simulink model "RealLifeTrainModel"  (R2024a)
settings: Solver=ode1  StartTime=0.0  StopTime=Inf  FixedStep=0.001  RelTol=1e-3
PostLoadFcn:
  | , if any(exist('dsrtsu_mdlpostloadfcn', 'file') ~= 0), dsrtsu_mdlpostloadfcn('Execute', bdroot); end,
InitFcn:
  | , if any(exist('rtifpga_mdlclblib', 'file') ~= 0), rtifpga_mdlclblib('Init', bdroot); end,
undefined symbols (not defined in the file): DiscIntNeverNeededParam
libraries: deeplib x29, svdutilitieslib x28, simulink x8, eeGeneralControl x8, rti1202lib_adc_class1 x6, rti1202serlib x5, spsEdgeDetectorLib x5, rtiemclib x2, rti1202lib_dac_class1 x1
(part 4 of 8)

== system RealLifeTrainModel/ContractionMetricFilterSystem3/Mdot_subsystem/IndidualGrad2 ==
  State : Inport
  Position : Inport  Port=2
  StartValue : Inport  Port=3
  ConvertMatrix : MATLAB Function  TreatAsAtomicUnit=on
  Data Type Conversion1 : DataTypeConversion  OutDataTypeStr=single  SaturateOnIntegerOverflow=off  RndMeth=Floor
  Data Type Conversion2 : DataTypeConversion  OutDataTypeStr=single  SaturateOnIntegerOverflow=off  RndMeth=Floor
  MATLAB Function2 : MATLAB Function  TreatAsAtomicUnit=on
  MATLAB Function5 : MATLAB Function  TreatAsAtomicUnit=on
  PredictMetric : deeplib/Predict  Network=Network from MAT-file  NetworkFunction=squeezenet  NetworkFilePath=C:\Users\ic2d\Documents\GitHub\dSpace_Controllers_legged\metric.mat  MiniBatchSize=128  InputDataFormats={'input', 'BC';}  Predictions=on  Activations={}  ForceInterpretedSim=off  EnableDLNetwork=on  LastKnownNetworkFilePath='C:\Users\ic2d\Documents\GitHub\dSpace_Controllers_legged\metric.mat'  LastKnownNetworkTimeStamp=739864.429490740760229527950286865234375
  Sum4 : Sum  Inputs=|++
  Grad : Outport
  wires:
  Sum4/1 -> Data Type Conversion2/1
  StartValue/1 -> MATLAB Function5/2(u2)
  Data Type Conversion1/1 -> ConvertMatrix/1(M_flat)
  [GradConst] -> MATLAB Function5/3(const)
  PredictMetric/1 -> Data Type Conversion1/1
  MATLAB Function5/1(y) -> Grad/1
  Position/1 -> MATLAB Function2/2(pos)
  [GradConst] -> MATLAB Function2/1(u)
  MATLAB Function2/1(y) -> Sum4/2
  State/1 -> Sum4/1
  Data Type Conversion2/1 -> PredictMetric/1
  ConvertMatrix/1(M) -> MATLAB Function5/1(u1)

== system RealLifeTrainModel/ContractionMetricFilterSystem3/Mdot_subsystem/IndidualGrad3 ==
  State : Inport
  Position : Inport  Port=2
  StartValue : Inport  Port=3
  ConvertMatrix : MATLAB Function  TreatAsAtomicUnit=on
  Data Type Conversion1 : DataTypeConversion  OutDataTypeStr=single  SaturateOnIntegerOverflow=off  RndMeth=Floor
  Data Type Conversion2 : DataTypeConversion  OutDataTypeStr=single  SaturateOnIntegerOverflow=off  RndMeth=Floor
  MATLAB Function2 : MATLAB Function  TreatAsAtomicUnit=on
  MATLAB Function5 : MATLAB Function  TreatAsAtomicUnit=on
  PredictMetric : deeplib/Predict  Network=Network from MAT-file  NetworkFunction=squeezenet  NetworkFilePath=C:\Users\ic2d\Documents\GitHub\dSpace_Controllers_legged\metric.mat  MiniBatchSize=128  InputDataFormats={'input', 'BC';}  Predictions=on  Activations={}  ForceInterpretedSim=off  EnableDLNetwork=on  LastKnownNetworkFilePath='C:\Users\ic2d\Documents\GitHub\dSpace_Controllers_legged\metric.mat'  LastKnownNetworkTimeStamp=739864.429490740760229527950286865234375
  Sum4 : Sum  Inputs=|++
  Grad : Outport
  wires:
  Sum4/1 -> Data Type Conversion2/1
  StartValue/1 -> MATLAB Function5/2(u2)
  Data Type Conversion1/1 -> ConvertMatrix/1(M_flat)
  [GradConst] -> MATLAB Function5/3(const)
  PredictMetric/1 -> Data Type Conversion1/1
  MATLAB Function5/1(y) -> Grad/1
  Position/1 -> MATLAB Function2/2(pos)
  [GradConst] -> MATLAB Function2/1(u)
  MATLAB Function2/1(y) -> Sum4/2
  State/1 -> Sum4/1
  Data Type Conversion2/1 -> PredictMetric/1
  ConvertMatrix/1(M) -> MATLAB Function5/1(u1)

== system RealLifeTrainModel/ContractionMetricFilterSystem3/Mdot_subsystem/IndidualGrad4 ==
  State : Inport
  Position : Inport  Port=2
  StartValue : Inport  Port=3
  ConvertMatrix : MATLAB Function  TreatAsAtomicUnit=on
  Data Type Conversion1 : DataTypeConversion  OutDataTypeStr=single  SaturateOnIntegerOverflow=off  RndMeth=Floor
  Data Type Conversion2 : DataTypeConversion  OutDataTypeStr=single  SaturateOnIntegerOverflow=off  RndMeth=Floor
  MATLAB Function2 : MATLAB Function  TreatAsAtomicUnit=on
  MATLAB Function5 : MATLAB Function  TreatAsAtomicUnit=on
  PredictMetric : deeplib/Predict  Network=Network from MAT-file  NetworkFunction=squeezenet  NetworkFilePath=C:\Users\ic2d\Documents\GitHub\dSpace_Controllers_legged\metric.mat  MiniBatchSize=128  InputDataFormats={'input', 'BC';}  Predictions=on  Activations={}  ForceInterpretedSim=off  EnableDLNetwork=on  LastKnownNetworkFilePath='C:\Users\ic2d\Documents\GitHub\dSpace_Controllers_legged\metric.mat'  LastKnownNetworkTimeStamp=739864.429490740760229527950286865234375
  Sum4 : Sum  Inputs=|++
  Grad : Outport
  wires:
  Sum4/1 -> Data Type Conversion2/1
  StartValue/1 -> MATLAB Function5/2(u2)
  Data Type Conversion1/1 -> ConvertMatrix/1(M_flat)
  [GradConst] -> MATLAB Function5/3(const)
  PredictMetric/1 -> Data Type Conversion1/1
  MATLAB Function5/1(y) -> Grad/1
  Position/1 -> MATLAB Function2/2(pos)
  [GradConst] -> MATLAB Function2/1(u)
  MATLAB Function2/1(y) -> Sum4/2
  State/1 -> Sum4/1
  Data Type Conversion2/1 -> PredictMetric/1
  ConvertMatrix/1(M) -> MATLAB Function5/1(u1)

== system RealLifeTrainModel/ContractionMetricFilterSystem3/Mdot_subsystem/IndidualGrad5 ==
  State : Inport
  Position : Inport  Port=2
  StartValue : Inport  Port=3
  ConvertMatrix : MATLAB Function  TreatAsAtomicUnit=on
  Data Type Conversion1 : DataTypeConversion  OutDataTypeStr=single  SaturateOnIntegerOverflow=off  RndMeth=Floor
  Data Type Conversion2 : DataTypeConversion  OutDataTypeStr=single  SaturateOnIntegerOverflow=off  RndMeth=Floor
  MATLAB Function2 : MATLAB Function  TreatAsAtomicUnit=on
  MATLAB Function5 : MATLAB Function  TreatAsAtomicUnit=on
  PredictMetric : deeplib/Predict  Network=Network from MAT-file  NetworkFunction=squeezenet  NetworkFilePath=C:\Users\ic2d\Documents\GitHub\dSpace_Controllers_legged\metric.mat  MiniBatchSize=128  InputDataFormats={'input', 'BC';}  Predictions=on  Activations={}  ForceInterpretedSim=off  EnableDLNetwork=on  LastKnownNetworkFilePath='C:\Users\ic2d\Documents\GitHub\dSpace_Controllers_legged\metric.mat'  LastKnownNetworkTimeStamp=739864.429490740760229527950286865234375
  Sum4 : Sum  Inputs=|++
  Grad : Outport
  wires:
  Sum4/1 -> Data Type Conversion2/1
  StartValue/1 -> MATLAB Function5/2(u2)
  Data Type Conversion1/1 -> ConvertMatrix/1(M_flat)
  [GradConst] -> MATLAB Function5/3(const)
  PredictMetric/1 -> Data Type Conversion1/1
  MATLAB Function5/1(y) -> Grad/1
  Position/1 -> MATLAB Function2/2(pos)
  [GradConst] -> MATLAB Function2/1(u)
  MATLAB Function2/1(y) -> Sum4/2
  State/1 -> Sum4/1
  Data Type Conversion2/1 -> PredictMetric/1
  ConvertMatrix/1(M) -> MATLAB Function5/1(u1)

== system RealLifeTrainModel/ContractionMetricFilterSystem3/Mdot_subsystem/IndidualGrad6 ==
  State : Inport
  Position : Inport  Port=2
  StartValue : Inport  Port=3
  ConvertMatrix : MATLAB Function  TreatAsAtomicUnit=on
  Data Type Conversion1 : DataTypeConversion  OutDataTypeStr=single  SaturateOnIntegerOverflow=off  RndMeth=Floor
  Data Type Conversion2 : DataTypeConversion  OutDataTypeStr=single  SaturateOnIntegerOverflow=off  RndMeth=Floor
  MATLAB Function2 : MATLAB Function  TreatAsAtomicUnit=on
  MATLAB Function5 : MATLAB Function  TreatAsAtomicUnit=on
  PredictMetric : deeplib/Predict  Network=Network from MAT-file  NetworkFunction=squeezenet  NetworkFilePath=C:\Users\ic2d\Documents\GitHub\dSpace_Controllers_legged\metric.mat  MiniBatchSize=128  InputDataFormats={'input', 'BC';}  Predictions=on  Activations={}  ForceInterpretedSim=off  EnableDLNetwork=on  LastKnownNetworkFilePath='C:\Users\ic2d\Documents\GitHub\dSpace_Controllers_legged\metric.mat'  LastKnownNetworkTimeStamp=739864.429490740760229527950286865234375
  Sum4 : Sum  Inputs=|++
  Grad : Outport
  wires:
  Sum4/1 -> Data Type Conversion2/1
  StartValue/1 -> MATLAB Function5/2(u2)
  Data Type Conversion1/1 -> ConvertMatrix/1(M_flat)
  [GradConst] -> MATLAB Function5/3(const)
  PredictMetric/1 -> Data Type Conversion1/1
  MATLAB Function5/1(y) -> Grad/1
  Position/1 -> MATLAB Function2/2(pos)
  [GradConst] -> MATLAB Function2/1(u)
  MATLAB Function2/1(y) -> Sum4/2
  State/1 -> Sum4/1
  Data Type Conversion2/1 -> PredictMetric/1
  ConvertMatrix/1(M) -> MATLAB Function5/1(u1)

== system RealLifeTrainModel/ContractionMetricFilterSystem3/Mdot_subsystem/IndidualGrad7 ==
  State : Inport
  Position : Inport  Port=2
  StartValue : Inport  Port=3
  ConvertMatrix : MATLAB Function  TreatAsAtomicUnit=on
  Data Type Conversion1 : DataTypeConversion  OutDataTypeStr=single  SaturateOnIntegerOverflow=off  RndMeth=Floor
  Data Type Conversion2 : DataTypeConversion  OutDataTypeStr=single  SaturateOnIntegerOverflow=off  RndMeth=Floor
  MATLAB Function2 : MATLAB Function  TreatAsAtomicUnit=on
  MATLAB Function5 : MATLAB Function  TreatAsAtomicUnit=on
  PredictMetric : deeplib/Predict  Network=Network from MAT-file  NetworkFunction=squeezenet  NetworkFilePath=C:\Users\ic2d\Documents\GitHub\dSpace_Controllers_legged\metric.mat  MiniBatchSize=128  InputDataFormats={'input', 'BC';}  Predictions=on  Activations={}  ForceInterpretedSim=off  EnableDLNetwork=on  LastKnownNetworkFilePath='C:\Users\ic2d\Documents\GitHub\dSpace_Controllers_legged\metric.mat'  LastKnownNetworkTimeStamp=739864.429490740760229527950286865234375
  Sum4 : Sum  Inputs=|++
  Grad : Outport
  wires:
  Sum4/1 -> Data Type Conversion2/1
  StartValue/1 -> MATLAB Function5/2(u2)
  Data Type Conversion1/1 -> ConvertMatrix/1(M_flat)
  [GradConst] -> MATLAB Function5/3(const)
  PredictMetric/1 -> Data Type Conversion1/1
  MATLAB Function5/1(y) -> Grad/1
  Position/1 -> MATLAB Function2/2(pos)
  [GradConst] -> MATLAB Function2/1(u)
  MATLAB Function2/1(y) -> Sum4/2
  State/1 -> Sum4/1
  Data Type Conversion2/1 -> PredictMetric/1
  ConvertMatrix/1(M) -> MATLAB Function5/1(u1)

== system RealLifeTrainModel/RTI Data/RTI Data Store/RTI Data Store ==
  RTI Data Store : Subsystem  mask(RTI_DATA_STORE){}
      mask help:
      | RTI Data Store Block. This block is used by RTI to store internal model dependent data. Deleting this block will result in data loss.
      |
      | NEVER DELETE, COPY, OR MODIFY THIS BLOCK!
      mask Help:
      | RTI Data Store Block. This block is used by RTI to store internal model dependent data. Deleting this block will result in data loss.
      | 
      | NEVER DELETE, COPY, OR MODIFY THIS BLOCK!
      mask Display: text(0.5, 0.5, ' ', 'HorizontalAlignment', 'center');

== system RealLifeTrainModel/CommSystem/SendMessageSystem/CancelSubsystem/If Action Subsystem ==
  Action Port : ActionPort  ActionPortLabel=if(u1 > 0)
  Cast : DataTypeConversion  OutDataTypeStr=double  SaturateOnIntegerOverflow=off  RndMeth=Floor
  Cast1 : DataTypeConversion  OutDataTypeStr=double  SaturateOnIntegerOverflow=off  RndMeth=Floor
  Constant : Constant  Value=0  OutDataTypeStr=uint8
  Data Store Write : DataStoreWrite  DataStoreName=FlagAbort  IndexOptions=Index vector (dialog)  Indices=1  OutputSizes=1
  Data Store Write2 : DataStoreWrite  DataStoreName=FlagStartTrain  IndexOptions=Index vector (dialog)  Indices=1  OutputSizes=1
  Data Store Write3 : DataStoreWrite  DataStoreName=OutputReceived  IndexOptions=Index vector (dialog)  Indices=1  OutputSizes=1
  Data Store Write4 : DataStoreWrite  DataStoreName=StartSignalValue  IndexOptions=Index vector (dialog)  Indices=1  OutputSizes=1
  wires:
  Constant/1 -> Cast1/1, Cast/1, Data Store Write2/1, Data Store Write/1
  Cast1/1 -> Data Store Write3/1
  Cast/1 -> Data Store Write4/1

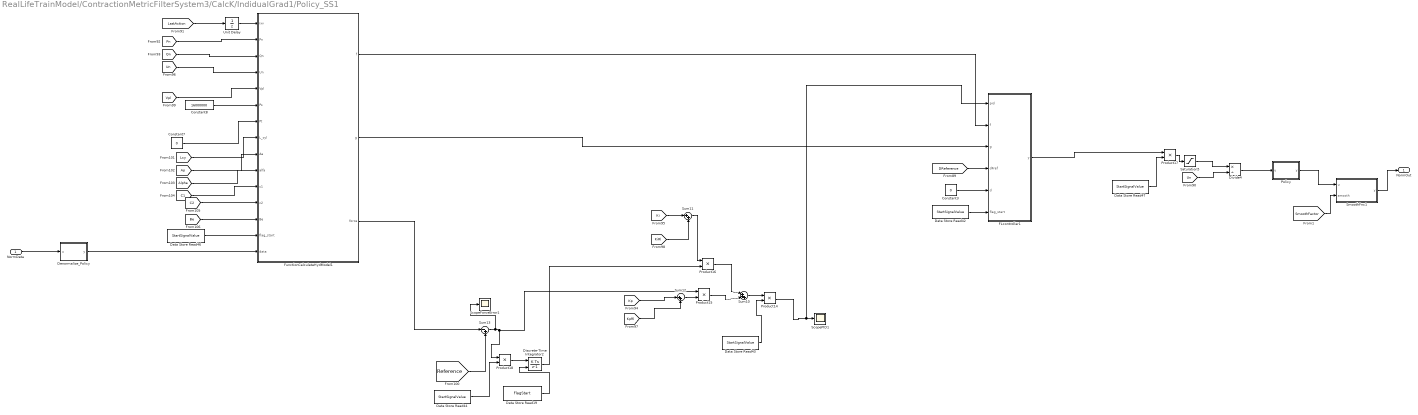
== system RealLifeTrainModel/ContractionMetricFilterSystem3/CalcK/IndidualGrad1/Policy_SS1 ==
  NormData : Inport
  Constant3 : Constant  Value=0
  Constant7 : Constant  Value=0
  Constant8 : Constant  Value=16000000
  Data Store Read19 : DataStoreRead  DataStoreName=FlagStart  IndexOptions=Index vector (dialog)  Indices=1  OutputSizes=1
  Data Store Read{42..44,46..47} (5 alike) : DataStoreRead  DataStoreName=StartSignalValue  IndexOptions=Index vector (dialog)  Indices=1  OutputSizes=1
  Denormalize_Policy : MATLAB Function  TreatAsAtomicUnit=on
  Discrete-Time Integrator2 : DiscreteIntegrator  ExternalReset=either  SampleTime=-1  ICPrevOutput=DiscIntNeverNeededParam  ICPrevScaledInput=DiscIntNeverNeededParam
  Divide4 : Product  Inputs=*/
  FLcontroller1 : MATLAB Function  TreatAsAtomicUnit=on
  FunctionCalculateHydModel1 : MATLAB Function  TreatAsAtomicUnit=on
  Policy : MATLAB Function  TreatAsAtomicUnit=on
  Product{14..18} (5 alike) : Product
  Saturation5 : Saturate  UpperLimit=str2num(get_param('Teste_PID/Un','Value'))/str2num(get_param('Teste_PID/SaturationDivider','Value'))  LowerLimit=-str2num(get_param('Teste_PID/Un','Value'))/str2num(get_param('Teste_PID/SaturationDivider','Value'))
  ScopeForceError1 : Scope
  ScopePID1 : Scope
  SmoothFnc1 : MATLAB Function  TreatAsAtomicUnit=on
  Sum10 : Sum  Inputs=|+++
  Sum11 : Sum  Inputs=|++
  Sum12 : Sum  Inputs=|++
  Sum13 : Sum  Inputs=|-+
  Unit Delay : UnitDelay  SampleTime=-1  HasFrameUpgradeWarning=on
  NormOut : Outport
  wires:
  FunctionCalculateHydModel1/3(force) -> Sum13/1
  [Vpl] -> FunctionCalculateHydModel1/5(Vpl)
  Sum13/1 -> ScopeForceError1/1, Product15/1, Product18/1
  [Alpha] -> FunctionCalculateHydModel1/10(alfa)
  [C2] -> FunctionCalculateHydModel1/12(c2)
  Data Store Read42/1 -> FLcontroller1/6(flag_start)
  [Be] -> FunctionCalculateHydModel1/13(Be)
  [Lcy] -> FunctionCalculateHydModel1/8(L_cyl)
  Data Store Read43/1 -> Product14/2
  [Ap] -> FunctionCalculateHydModel1/9(Aa)
  Product15/1 -> Sum10/2
  Data Store Read44/1 -> Product18/2
  Product18/1 -> Discrete-Time Integrator2/1
  [KpRl] -> Sum12/2
  [Reference] -> Sum13/2
  Constant8/1 -> FunctionCalculateHydModel1/6(Ps)
  Product14/1 -> FLcontroller1/1(pid), ScopePID1/1
  Sum11/1 -> Product16/1
  Sum12/1 -> Product15/2
  Saturation5/1 -> Divide4/1
  [Un] -> Divide4/2
  FLcontroller1/1(y) -> Product17/1
  Denormalize_Policy/1(y) -> FunctionCalculateHydModel1/15(data)
  Sum10/1 -> Product14/1
  [C1] -> FunctionCalculateHydModel1/11(c1)
  Discrete-Time Integrator2/1 -> Product16/2
  [Pn] -> FunctionCalculateHydModel1/2(Pn)
  [LastAction] -> Unit Delay/1
  [Kp] -> Sum12/1
  [Ki] -> Sum11/1
  Constant7/1 -> FunctionCalculateHydModel1/7(Pt)
  Divide4/1 -> Policy/1(u)
  [Qn] -> FunctionCalculateHydModel1/3(Qn)
  Constant3/1 -> FLcontroller1/5(d)
  [KiRl] -> Sum11/2
  Data Store Read47/1 -> Product17/2
  Product16/1 -> Sum10/1
  FunctionCalculateHydModel1/2(g) -> FLcontroller1/3(g)
  Product17/1 -> Saturation5/1
  [DReference] -> FLcontroller1/4(dFref)
  FunctionCalculateHydModel1/1(f) -> FLcontroller1/2(f)
  [Un] -> FunctionCalculateHydModel1/4(Un)
  Data Store Read46/1 -> FunctionCalculateHydModel1/14(flag_start)
  NormData/1 -> Denormalize_Policy/1(u)
  Unit Delay/1 -> FunctionCalculateHydModel1/1(ixv)
  SmoothFnc1/1(y) -> NormOut/1
  Policy/1(y) -> SmoothFnc1/1(u)
  [SmoothFactor] -> SmoothFnc1/2(smooth)
  Data Store Read19/1 -> Discrete-Time Integrator2/2

== system RealLifeTrainModel/ContractionMetricFilterSystem3/CalcK/IndidualGrad10/Policy_SS1 ==
  NormData : Inport
  Constant3 : Constant  Value=0
  Constant7 : Constant  Value=0
  Constant8 : Constant  Value=16000000
  Data Store Read19 : DataStoreRead  DataStoreName=FlagStart  IndexOptions=Index vector (dialog)  Indices=1  OutputSizes=1
  Data Store Read{42..44,46..47} (5 alike) : DataStoreRead  DataStoreName=StartSignalValue  IndexOptions=Index vector (dialog)  Indices=1  OutputSizes=1
  Denormalize_Policy : MATLAB Function  TreatAsAtomicUnit=on
  Discrete-Time Integrator2 : DiscreteIntegrator  ExternalReset=either  SampleTime=-1  ICPrevOutput=DiscIntNeverNeededParam  ICPrevScaledInput=DiscIntNeverNeededParam
  Divide4 : Product  Inputs=*/
  FLcontroller1 : MATLAB Function  TreatAsAtomicUnit=on
  FunctionCalculateHydModel1 : MATLAB Function  TreatAsAtomicUnit=on
  Policy : MATLAB Function  TreatAsAtomicUnit=on
  Product{14..18} (5 alike) : Product
  Saturation5 : Saturate  UpperLimit=str2num(get_param('Teste_PID/Un','Value'))/str2num(get_param('Teste_PID/SaturationDivider','Value'))  LowerLimit=-str2num(get_param('Teste_PID/Un','Value'))/str2num(get_param('Teste_PID/SaturationDivider','Value'))
  ScopeForceError1 : Scope
  ScopePID1 : Scope
  SmoothFnc1 : MATLAB Function  TreatAsAtomicUnit=on
  Sum10 : Sum  Inputs=|+++
  Sum11 : Sum  Inputs=|++
  Sum12 : Sum  Inputs=|++
  Sum13 : Sum  Inputs=|-+
  Unit Delay : UnitDelay  SampleTime=-1  HasFrameUpgradeWarning=on
  NormOut : Outport
  wires:
  FunctionCalculateHydModel1/3(force) -> Sum13/1
  [Vpl] -> FunctionCalculateHydModel1/5(Vpl)
  Sum13/1 -> ScopeForceError1/1, Product15/1, Product18/1
  [Alpha] -> FunctionCalculateHydModel1/10(alfa)
  [C2] -> FunctionCalculateHydModel1/12(c2)
  Data Store Read42/1 -> FLcontroller1/6(flag_start)
  [Be] -> FunctionCalculateHydModel1/13(Be)
  [Lcy] -> FunctionCalculateHydModel1/8(L_cyl)
  Data Store Read43/1 -> Product14/2
  [Ap] -> FunctionCalculateHydModel1/9(Aa)
  Product15/1 -> Sum10/2
  Data Store Read44/1 -> Product18/2
  Product18/1 -> Discrete-Time Integrator2/1
  [KpRl] -> Sum12/2
  [Reference] -> Sum13/2
  Constant8/1 -> FunctionCalculateHydModel1/6(Ps)
  Product14/1 -> FLcontroller1/1(pid), ScopePID1/1
  Sum11/1 -> Product16/1
  Sum12/1 -> Product15/2
  Saturation5/1 -> Divide4/1
  [Un] -> Divide4/2
  FLcontroller1/1(y) -> Product17/1
  Denormalize_Policy/1(y) -> FunctionCalculateHydModel1/15(data)
  Sum10/1 -> Product14/1
  [C1] -> FunctionCalculateHydModel1/11(c1)
  Discrete-Time Integrator2/1 -> Product16/2
  [Pn] -> FunctionCalculateHydModel1/2(Pn)
  [LastAction] -> Unit Delay/1
  [Kp] -> Sum12/1
  [Ki] -> Sum11/1
  Constant7/1 -> FunctionCalculateHydModel1/7(Pt)
  Divide4/1 -> Policy/1(u)
  [Qn] -> FunctionCalculateHydModel1/3(Qn)
  Constant3/1 -> FLcontroller1/5(d)
  [KiRl] -> Sum11/2
  Data Store Read47/1 -> Product17/2
  Product16/1 -> Sum10/1
  FunctionCalculateHydModel1/2(g) -> FLcontroller1/3(g)
  Product17/1 -> Saturation5/1
  [DReference] -> FLcontroller1/4(dFref)
  FunctionCalculateHydModel1/1(f) -> FLcontroller1/2(f)
  [Un] -> FunctionCalculateHydModel1/4(Un)
  Data Store Read46/1 -> FunctionCalculateHydModel1/14(flag_start)
  NormData/1 -> Denormalize_Policy/1(u)
  Unit Delay/1 -> FunctionCalculateHydModel1/1(ixv)
  SmoothFnc1/1(y) -> NormOut/1
  Policy/1(y) -> SmoothFnc1/1(u)
  [SmoothFactor] -> SmoothFnc1/2(smooth)
  Data Store Read19/1 -> Discrete-Time Integrator2/2

== system RealLifeTrainModel/ContractionMetricFilterSystem3/CalcK/IndidualGrad2/Policy_SS1 ==
  NormData : Inport
  Constant3 : Constant  Value=0
  Constant7 : Constant  Value=0
  Constant8 : Constant  Value=16000000
  Data Store Read19 : DataStoreRead  DataStoreName=FlagStart  IndexOptions=Index vector (dialog)  Indices=1  OutputSizes=1
  Data Store Read{42..44,46..47} (5 alike) : DataStoreRead  DataStoreName=StartSignalValue  IndexOptions=Index vector (dialog)  Indices=1  OutputSizes=1
  Denormalize_Policy : MATLAB Function  TreatAsAtomicUnit=on
  Discrete-Time Integrator2 : DiscreteIntegrator  ExternalReset=either  SampleTime=-1  ICPrevOutput=DiscIntNeverNeededParam  ICPrevScaledInput=DiscIntNeverNeededParam
  Divide4 : Product  Inputs=*/
  FLcontroller1 : MATLAB Function  TreatAsAtomicUnit=on
  FunctionCalculateHydModel1 : MATLAB Function  TreatAsAtomicUnit=on
  Policy : MATLAB Function  TreatAsAtomicUnit=on
  Product{14..18} (5 alike) : Product
  Saturation5 : Saturate  UpperLimit=str2num(get_param('Teste_PID/Un','Value'))/str2num(get_param('Teste_PID/SaturationDivider','Value'))  LowerLimit=-str2num(get_param('Teste_PID/Un','Value'))/str2num(get_param('Teste_PID/SaturationDivider','Value'))
  ScopeForceError1 : Scope
  ScopePID1 : Scope
  SmoothFnc1 : MATLAB Function  TreatAsAtomicUnit=on
  Sum10 : Sum  Inputs=|+++
  Sum11 : Sum  Inputs=|++
  Sum12 : Sum  Inputs=|++
  Sum13 : Sum  Inputs=|-+
  Unit Delay : UnitDelay  SampleTime=-1  HasFrameUpgradeWarning=on
  NormOut : Outport
  wires:
  FunctionCalculateHydModel1/3(force) -> Sum13/1
  [Vpl] -> FunctionCalculateHydModel1/5(Vpl)
  Sum13/1 -> ScopeForceError1/1, Product15/1, Product18/1
  [Alpha] -> FunctionCalculateHydModel1/10(alfa)
  [C2] -> FunctionCalculateHydModel1/12(c2)
  Data Store Read42/1 -> FLcontroller1/6(flag_start)
  [Be] -> FunctionCalculateHydModel1/13(Be)
  [Lcy] -> FunctionCalculateHydModel1/8(L_cyl)
  Data Store Read43/1 -> Product14/2
  [Ap] -> FunctionCalculateHydModel1/9(Aa)
  Product15/1 -> Sum10/2
  Data Store Read44/1 -> Product18/2
  Product18/1 -> Discrete-Time Integrator2/1
  [KpRl] -> Sum12/2
  [Reference] -> Sum13/2
  Constant8/1 -> FunctionCalculateHydModel1/6(Ps)
  Product14/1 -> FLcontroller1/1(pid), ScopePID1/1
  Sum11/1 -> Product16/1
  Sum12/1 -> Product15/2
  Saturation5/1 -> Divide4/1
  [Un] -> Divide4/2
  FLcontroller1/1(y) -> Product17/1
  Denormalize_Policy/1(y) -> FunctionCalculateHydModel1/15(data)
  Sum10/1 -> Product14/1
  [C1] -> FunctionCalculateHydModel1/11(c1)
  Discrete-Time Integrator2/1 -> Product16/2
  [Pn] -> FunctionCalculateHydModel1/2(Pn)
  [LastAction] -> Unit Delay/1
  [Kp] -> Sum12/1
  [Ki] -> Sum11/1
  Constant7/1 -> FunctionCalculateHydModel1/7(Pt)
  Divide4/1 -> Policy/1(u)
  [Qn] -> FunctionCalculateHydModel1/3(Qn)
  Constant3/1 -> FLcontroller1/5(d)
  [KiRl] -> Sum11/2
  Data Store Read47/1 -> Product17/2
  Product16/1 -> Sum10/1
  FunctionCalculateHydModel1/2(g) -> FLcontroller1/3(g)
  Product17/1 -> Saturation5/1
  [DReference] -> FLcontroller1/4(dFref)
  FunctionCalculateHydModel1/1(f) -> FLcontroller1/2(f)
  [Un] -> FunctionCalculateHydModel1/4(Un)
  Data Store Read46/1 -> FunctionCalculateHydModel1/14(flag_start)
  NormData/1 -> Denormalize_Policy/1(u)
  Unit Delay/1 -> FunctionCalculateHydModel1/1(ixv)
  SmoothFnc1/1(y) -> NormOut/1
  Policy/1(y) -> SmoothFnc1/1(u)
  [SmoothFactor] -> SmoothFnc1/2(smooth)
  Data Store Read19/1 -> Discrete-Time Integrator2/2

== system RealLifeTrainModel/ContractionMetricFilterSystem3/CalcK/IndidualGrad3/Policy_SS1 ==
  NormData : Inport
  Constant3 : Constant  Value=0
  Constant7 : Constant  Value=0
  Constant8 : Constant  Value=16000000
  Data Store Read19 : DataStoreRead  DataStoreName=FlagStart  IndexOptions=Index vector (dialog)  Indices=1  OutputSizes=1
  Data Store Read{42..44,46..47} (5 alike) : DataStoreRead  DataStoreName=StartSignalValue  IndexOptions=Index vector (dialog)  Indices=1  OutputSizes=1
  Denormalize_Policy : MATLAB Function  TreatAsAtomicUnit=on
  Discrete-Time Integrator2 : DiscreteIntegrator  ExternalReset=either  SampleTime=-1  ICPrevOutput=DiscIntNeverNeededParam  ICPrevScaledInput=DiscIntNeverNeededParam
  Divide4 : Product  Inputs=*/
  FLcontroller1 : MATLAB Function  TreatAsAtomicUnit=on
  FunctionCalculateHydModel1 : MATLAB Function  TreatAsAtomicUnit=on
  Policy : MATLAB Function  TreatAsAtomicUnit=on
  Product{14..18} (5 alike) : Product
  Saturation5 : Saturate  UpperLimit=str2num(get_param('Teste_PID/Un','Value'))/str2num(get_param('Teste_PID/SaturationDivider','Value'))  LowerLimit=-str2num(get_param('Teste_PID/Un','Value'))/str2num(get_param('Teste_PID/SaturationDivider','Value'))
  ScopeForceError1 : Scope
  ScopePID1 : Scope
  SmoothFnc1 : MATLAB Function  TreatAsAtomicUnit=on
  Sum10 : Sum  Inputs=|+++
  Sum11 : Sum  Inputs=|++
  Sum12 : Sum  Inputs=|++
  Sum13 : Sum  Inputs=|-+
  Unit Delay : UnitDelay  SampleTime=-1  HasFrameUpgradeWarning=on
  NormOut : Outport
  wires:
  FunctionCalculateHydModel1/3(force) -> Sum13/1
  [Vpl] -> FunctionCalculateHydModel1/5(Vpl)
  Sum13/1 -> ScopeForceError1/1, Product15/1, Product18/1
  [Alpha] -> FunctionCalculateHydModel1/10(alfa)
  [C2] -> FunctionCalculateHydModel1/12(c2)
  Data Store Read42/1 -> FLcontroller1/6(flag_start)
  [Be] -> FunctionCalculateHydModel1/13(Be)
  [Lcy] -> FunctionCalculateHydModel1/8(L_cyl)
  Data Store Read43/1 -> Product14/2
  [Ap] -> FunctionCalculateHydModel1/9(Aa)
  Product15/1 -> Sum10/2
  Data Store Read44/1 -> Product18/2
  Product18/1 -> Discrete-Time Integrator2/1
  [KpRl] -> Sum12/2
  [Reference] -> Sum13/2
  Constant8/1 -> FunctionCalculateHydModel1/6(Ps)
  Product14/1 -> FLcontroller1/1(pid), ScopePID1/1
  Sum11/1 -> Product16/1
  Sum12/1 -> Product15/2
  Saturation5/1 -> Divide4/1
  [Un] -> Divide4/2
  FLcontroller1/1(y) -> Product17/1
  Denormalize_Policy/1(y) -> FunctionCalculateHydModel1/15(data)
  Sum10/1 -> Product14/1
  [C1] -> FunctionCalculateHydModel1/11(c1)
  Discrete-Time Integrator2/1 -> Product16/2
  [Pn] -> FunctionCalculateHydModel1/2(Pn)
  [LastAction] -> Unit Delay/1
  [Kp] -> Sum12/1
  [Ki] -> Sum11/1
  Constant7/1 -> FunctionCalculateHydModel1/7(Pt)
  Divide4/1 -> Policy/1(u)
  [Qn] -> FunctionCalculateHydModel1/3(Qn)
  Constant3/1 -> FLcontroller1/5(d)
  [KiRl] -> Sum11/2
  Data Store Read47/1 -> Product17/2
  Product16/1 -> Sum10/1
  FunctionCalculateHydModel1/2(g) -> FLcontroller1/3(g)
  Product17/1 -> Saturation5/1
  [DReference] -> FLcontroller1/4(dFref)
  FunctionCalculateHydModel1/1(f) -> FLcontroller1/2(f)
  [Un] -> FunctionCalculateHydModel1/4(Un)
  Data Store Read46/1 -> FunctionCalculateHydModel1/14(flag_start)
  NormData/1 -> Denormalize_Policy/1(u)
  Unit Delay/1 -> FunctionCalculateHydModel1/1(ixv)
  SmoothFnc1/1(y) -> NormOut/1
  Policy/1(y) -> SmoothFnc1/1(u)
  [SmoothFactor] -> SmoothFnc1/2(smooth)
  Data Store Read19/1 -> Discrete-Time Integrator2/2

== system RealLifeTrainModel/ContractionMetricFilterSystem3/CalcK/IndidualGrad4/Policy_SS1 ==
  NormData : Inport
  Constant3 : Constant  Value=0
  Constant7 : Constant  Value=0
  Constant8 : Constant  Value=16000000
  Data Store Read19 : DataStoreRead  DataStoreName=FlagStart  IndexOptions=Index vector (dialog)  Indices=1  OutputSizes=1
  Data Store Read{42..44,46..47} (5 alike) : DataStoreRead  DataStoreName=StartSignalValue  IndexOptions=Index vector (dialog)  Indices=1  OutputSizes=1
  Denormalize_Policy : MATLAB Function  TreatAsAtomicUnit=on
  Discrete-Time Integrator2 : DiscreteIntegrator  ExternalReset=either  SampleTime=-1  ICPrevOutput=DiscIntNeverNeededParam  ICPrevScaledInput=DiscIntNeverNeededParam
  Divide4 : Product  Inputs=*/
  FLcontroller1 : MATLAB Function  TreatAsAtomicUnit=on
  FunctionCalculateHydModel1 : MATLAB Function  TreatAsAtomicUnit=on
  Policy : MATLAB Function  TreatAsAtomicUnit=on
  Product{14..18} (5 alike) : Product
  Saturation5 : Saturate  UpperLimit=str2num(get_param('Teste_PID/Un','Value'))/str2num(get_param('Teste_PID/SaturationDivider','Value'))  LowerLimit=-str2num(get_param('Teste_PID/Un','Value'))/str2num(get_param('Teste_PID/SaturationDivider','Value'))
  ScopeForceError1 : Scope
  ScopePID1 : Scope
  SmoothFnc1 : MATLAB Function  TreatAsAtomicUnit=on
  Sum10 : Sum  Inputs=|+++
  Sum11 : Sum  Inputs=|++
  Sum12 : Sum  Inputs=|++
  Sum13 : Sum  Inputs=|-+
  Unit Delay : UnitDelay  SampleTime=-1  HasFrameUpgradeWarning=on
  NormOut : Outport
  wires:
  FunctionCalculateHydModel1/3(force) -> Sum13/1
  [Vpl] -> FunctionCalculateHydModel1/5(Vpl)
  Sum13/1 -> ScopeForceError1/1, Product15/1, Product18/1
  [Alpha] -> FunctionCalculateHydModel1/10(alfa)
  [C2] -> FunctionCalculateHydModel1/12(c2)
  Data Store Read42/1 -> FLcontroller1/6(flag_start)
  [Be] -> FunctionCalculateHydModel1/13(Be)
  [Lcy] -> FunctionCalculateHydModel1/8(L_cyl)
  Data Store Read43/1 -> Product14/2
  [Ap] -> FunctionCalculateHydModel1/9(Aa)
  Product15/1 -> Sum10/2
  Data Store Read44/1 -> Product18/2
  Product18/1 -> Discrete-Time Integrator2/1
  [KpRl] -> Sum12/2
  [Reference] -> Sum13/2
  Constant8/1 -> FunctionCalculateHydModel1/6(Ps)
  Product14/1 -> FLcontroller1/1(pid), ScopePID1/1
  Sum11/1 -> Product16/1
  Sum12/1 -> Product15/2
  Saturation5/1 -> Divide4/1
  [Un] -> Divide4/2
  FLcontroller1/1(y) -> Product17/1
  Denormalize_Policy/1(y) -> FunctionCalculateHydModel1/15(data)
  Sum10/1 -> Product14/1
  [C1] -> FunctionCalculateHydModel1/11(c1)
  Discrete-Time Integrator2/1 -> Product16/2
  [Pn] -> FunctionCalculateHydModel1/2(Pn)
  [LastAction] -> Unit Delay/1
  [Kp] -> Sum12/1
  [Ki] -> Sum11/1
  Constant7/1 -> FunctionCalculateHydModel1/7(Pt)
  Divide4/1 -> Policy/1(u)
  [Qn] -> FunctionCalculateHydModel1/3(Qn)
  Constant3/1 -> FLcontroller1/5(d)
  [KiRl] -> Sum11/2
  Data Store Read47/1 -> Product17/2
  Product16/1 -> Sum10/1
  FunctionCalculateHydModel1/2(g) -> FLcontroller1/3(g)
  Product17/1 -> Saturation5/1
  [DReference] -> FLcontroller1/4(dFref)
  FunctionCalculateHydModel1/1(f) -> FLcontroller1/2(f)
  [Un] -> FunctionCalculateHydModel1/4(Un)
  Data Store Read46/1 -> FunctionCalculateHydModel1/14(flag_start)
  NormData/1 -> Denormalize_Policy/1(u)
  Unit Delay/1 -> FunctionCalculateHydModel1/1(ixv)
  SmoothFnc1/1(y) -> NormOut/1
  Policy/1(y) -> SmoothFnc1/1(u)
  [SmoothFactor] -> SmoothFnc1/2(smooth)
  Data Store Read19/1 -> Discrete-Time Integrator2/2

== system RealLifeTrainModel/ContractionMetricFilterSystem3/CalcK/IndidualGrad5/Policy_SS1 ==
  NormData : Inport
  Constant3 : Constant  Value=0
  Constant7 : Constant  Value=0
  Constant8 : Constant  Value=16000000
  Data Store Read19 : DataStoreRead  DataStoreName=FlagStart  IndexOptions=Index vector (dialog)  Indices=1  OutputSizes=1
  Data Store Read{42..44,46..47} (5 alike) : DataStoreRead  DataStoreName=StartSignalValue  IndexOptions=Index vector (dialog)  Indices=1  OutputSizes=1
  Denormalize_Policy : MATLAB Function  TreatAsAtomicUnit=on
  Discrete-Time Integrator2 : DiscreteIntegrator  ExternalReset=either  SampleTime=-1  ICPrevOutput=DiscIntNeverNeededParam  ICPrevScaledInput=DiscIntNeverNeededParam
  Divide4 : Product  Inputs=*/
  FLcontroller1 : MATLAB Function  TreatAsAtomicUnit=on
  FunctionCalculateHydModel1 : MATLAB Function  TreatAsAtomicUnit=on
  Policy : MATLAB Function  TreatAsAtomicUnit=on
  Product{14..18} (5 alike) : Product
  Saturation5 : Saturate  UpperLimit=str2num(get_param('Teste_PID/Un','Value'))/str2num(get_param('Teste_PID/SaturationDivider','Value'))  LowerLimit=-str2num(get_param('Teste_PID/Un','Value'))/str2num(get_param('Teste_PID/SaturationDivider','Value'))
  ScopeForceError1 : Scope
  ScopePID1 : Scope
  SmoothFnc1 : MATLAB Function  TreatAsAtomicUnit=on
  Sum10 : Sum  Inputs=|+++
  Sum11 : Sum  Inputs=|++
  Sum12 : Sum  Inputs=|++
  Sum13 : Sum  Inputs=|-+
  Unit Delay : UnitDelay  SampleTime=-1  HasFrameUpgradeWarning=on
  NormOut : Outport
  wires:
  FunctionCalculateHydModel1/3(force) -> Sum13/1
  [Vpl] -> FunctionCalculateHydModel1/5(Vpl)
  Sum13/1 -> ScopeForceError1/1, Product15/1, Product18/1
  [Alpha] -> FunctionCalculateHydModel1/10(alfa)
  [C2] -> FunctionCalculateHydModel1/12(c2)
  Data Store Read42/1 -> FLcontroller1/6(flag_start)
  [Be] -> FunctionCalculateHydModel1/13(Be)
  [Lcy] -> FunctionCalculateHydModel1/8(L_cyl)
  Data Store Read43/1 -> Product14/2
  [Ap] -> FunctionCalculateHydModel1/9(Aa)
  Product15/1 -> Sum10/2
  Data Store Read44/1 -> Product18/2
  Product18/1 -> Discrete-Time Integrator2/1
  [KpRl] -> Sum12/2
  [Reference] -> Sum13/2
  Constant8/1 -> FunctionCalculateHydModel1/6(Ps)
  Product14/1 -> FLcontroller1/1(pid), ScopePID1/1
  Sum11/1 -> Product16/1
  Sum12/1 -> Product15/2
  Saturation5/1 -> Divide4/1
  [Un] -> Divide4/2
  FLcontroller1/1(y) -> Product17/1
  Denormalize_Policy/1(y) -> FunctionCalculateHydModel1/15(data)
  Sum10/1 -> Product14/1
  [C1] -> FunctionCalculateHydModel1/11(c1)
  Discrete-Time Integrator2/1 -> Product16/2
  [Pn] -> FunctionCalculateHydModel1/2(Pn)
  [LastAction] -> Unit Delay/1
  [Kp] -> Sum12/1
  [Ki] -> Sum11/1
  Constant7/1 -> FunctionCalculateHydModel1/7(Pt)
  Divide4/1 -> Policy/1(u)
  [Qn] -> FunctionCalculateHydModel1/3(Qn)
  Constant3/1 -> FLcontroller1/5(d)
  [KiRl] -> Sum11/2
  Data Store Read47/1 -> Product17/2
  Product16/1 -> Sum10/1
  FunctionCalculateHydModel1/2(g) -> FLcontroller1/3(g)
  Product17/1 -> Saturation5/1
  [DReference] -> FLcontroller1/4(dFref)
  FunctionCalculateHydModel1/1(f) -> FLcontroller1/2(f)
  [Un] -> FunctionCalculateHydModel1/4(Un)
  Data Store Read46/1 -> FunctionCalculateHydModel1/14(flag_start)
  NormData/1 -> Denormalize_Policy/1(u)
  Unit Delay/1 -> FunctionCalculateHydModel1/1(ixv)
  SmoothFnc1/1(y) -> NormOut/1
  Policy/1(y) -> SmoothFnc1/1(u)
  [SmoothFactor] -> SmoothFnc1/2(smooth)
  Data Store Read19/1 -> Discrete-Time Integrator2/2

== system RealLifeTrainModel/ContractionMetricFilterSystem3/CalcK/IndidualGrad6/Policy_SS1 ==
  NormData : Inport
  Constant3 : Constant  Value=0
  Constant7 : Constant  Value=0
  Constant8 : Constant  Value=16000000
  Data Store Read19 : DataStoreRead  DataStoreName=FlagStart  IndexOptions=Index vector (dialog)  Indices=1  OutputSizes=1
  Data Store Read{42..44,46..47} (5 alike) : DataStoreRead  DataStoreName=StartSignalValue  IndexOptions=Index vector (dialog)  Indices=1  OutputSizes=1
  Denormalize_Policy : MATLAB Function  TreatAsAtomicUnit=on
  Discrete-Time Integrator2 : DiscreteIntegrator  ExternalReset=either  SampleTime=-1  ICPrevOutput=DiscIntNeverNeededParam  ICPrevScaledInput=DiscIntNeverNeededParam
  Divide4 : Product  Inputs=*/
  FLcontroller1 : MATLAB Function  TreatAsAtomicUnit=on
  FunctionCalculateHydModel1 : MATLAB Function  TreatAsAtomicUnit=on
  Policy : MATLAB Function  TreatAsAtomicUnit=on
  Product{14..18} (5 alike) : Product
  Saturation5 : Saturate  UpperLimit=str2num(get_param('Teste_PID/Un','Value'))/str2num(get_param('Teste_PID/SaturationDivider','Value'))  LowerLimit=-str2num(get_param('Teste_PID/Un','Value'))/str2num(get_param('Teste_PID/SaturationDivider','Value'))
  ScopeForceError1 : Scope
  ScopePID1 : Scope
  SmoothFnc1 : MATLAB Function  TreatAsAtomicUnit=on
  Sum10 : Sum  Inputs=|+++
  Sum11 : Sum  Inputs=|++
  Sum12 : Sum  Inputs=|++
  Sum13 : Sum  Inputs=|-+
  Unit Delay : UnitDelay  SampleTime=-1  HasFrameUpgradeWarning=on
  NormOut : Outport
  wires:
  FunctionCalculateHydModel1/3(force) -> Sum13/1
  [Vpl] -> FunctionCalculateHydModel1/5(Vpl)
  Sum13/1 -> ScopeForceError1/1, Product15/1, Product18/1
  [Alpha] -> FunctionCalculateHydModel1/10(alfa)
  [C2] -> FunctionCalculateHydModel1/12(c2)
  Data Store Read42/1 -> FLcontroller1/6(flag_start)
  [Be] -> FunctionCalculateHydModel1/13(Be)
  [Lcy] -> FunctionCalculateHydModel1/8(L_cyl)
  Data Store Read43/1 -> Product14/2
  [Ap] -> FunctionCalculateHydModel1/9(Aa)
  Product15/1 -> Sum10/2
  Data Store Read44/1 -> Product18/2
  Product18/1 -> Discrete-Time Integrator2/1
  [KpRl] -> Sum12/2
  [Reference] -> Sum13/2
  Constant8/1 -> FunctionCalculateHydModel1/6(Ps)
  Product14/1 -> FLcontroller1/1(pid), ScopePID1/1
  Sum11/1 -> Product16/1
  Sum12/1 -> Product15/2
  Saturation5/1 -> Divide4/1
  [Un] -> Divide4/2
  FLcontroller1/1(y) -> Product17/1
  Denormalize_Policy/1(y) -> FunctionCalculateHydModel1/15(data)
  Sum10/1 -> Product14/1
  [C1] -> FunctionCalculateHydModel1/11(c1)
  Discrete-Time Integrator2/1 -> Product16/2
  [Pn] -> FunctionCalculateHydModel1/2(Pn)
  [LastAction] -> Unit Delay/1
  [Kp] -> Sum12/1
  [Ki] -> Sum11/1
  Constant7/1 -> FunctionCalculateHydModel1/7(Pt)
  Divide4/1 -> Policy/1(u)
  [Qn] -> FunctionCalculateHydModel1/3(Qn)
  Constant3/1 -> FLcontroller1/5(d)
  [KiRl] -> Sum11/2
  Data Store Read47/1 -> Product17/2
  Product16/1 -> Sum10/1
  FunctionCalculateHydModel1/2(g) -> FLcontroller1/3(g)
  Product17/1 -> Saturation5/1
  [DReference] -> FLcontroller1/4(dFref)
  FunctionCalculateHydModel1/1(f) -> FLcontroller1/2(f)
  [Un] -> FunctionCalculateHydModel1/4(Un)
  Data Store Read46/1 -> FunctionCalculateHydModel1/14(flag_start)
  NormData/1 -> Denormalize_Policy/1(u)
  Unit Delay/1 -> FunctionCalculateHydModel1/1(ixv)
  SmoothFnc1/1(y) -> NormOut/1
  Policy/1(y) -> SmoothFnc1/1(u)
  [SmoothFactor] -> SmoothFnc1/2(smooth)
  Data Store Read19/1 -> Discrete-Time Integrator2/2

== system RealLifeTrainModel/ContractionMetricFilterSystem3/CalcK/IndidualGrad7/Policy_SS1 ==
  NormData : Inport
  Constant3 : Constant  Value=0
  Constant7 : Constant  Value=0
  Constant8 : Constant  Value=16000000
  Data Store Read19 : DataStoreRead  DataStoreName=FlagStart  IndexOptions=Index vector (dialog)  Indices=1  OutputSizes=1
  Data Store Read{42..44,46..47} (5 alike) : DataStoreRead  DataStoreName=StartSignalValue  IndexOptions=Index vector (dialog)  Indices=1  OutputSizes=1
  Denormalize_Policy : MATLAB Function  TreatAsAtomicUnit=on
  Discrete-Time Integrator2 : DiscreteIntegrator  ExternalReset=either  SampleTime=-1  ICPrevOutput=DiscIntNeverNeededParam  ICPrevScaledInput=DiscIntNeverNeededParam
  Divide4 : Product  Inputs=*/
  FLcontroller1 : MATLAB Function  TreatAsAtomicUnit=on
  FunctionCalculateHydModel1 : MATLAB Function  TreatAsAtomicUnit=on
  Policy : MATLAB Function  TreatAsAtomicUnit=on
  Product{14..18} (5 alike) : Product
  Saturation5 : Saturate  UpperLimit=str2num(get_param('Teste_PID/Un','Value'))/str2num(get_param('Teste_PID/SaturationDivider','Value'))  LowerLimit=-str2num(get_param('Teste_PID/Un','Value'))/str2num(get_param('Teste_PID/SaturationDivider','Value'))
  ScopeForceError1 : Scope
  ScopePID1 : Scope
  SmoothFnc1 : MATLAB Function  TreatAsAtomicUnit=on
  Sum10 : Sum  Inputs=|+++
  Sum11 : Sum  Inputs=|++
  Sum12 : Sum  Inputs=|++
  Sum13 : Sum  Inputs=|-+
  Unit Delay : UnitDelay  SampleTime=-1  HasFrameUpgradeWarning=on
  NormOut : Outport
  wires:
  FunctionCalculateHydModel1/3(force) -> Sum13/1
  [Vpl] -> FunctionCalculateHydModel1/5(Vpl)
  Sum13/1 -> ScopeForceError1/1, Product15/1, Product18/1
  [Alpha] -> FunctionCalculateHydModel1/10(alfa)
  [C2] -> FunctionCalculateHydModel1/12(c2)
  Data Store Read42/1 -> FLcontroller1/6(flag_start)
  [Be] -> FunctionCalculateHydModel1/13(Be)
  [Lcy] -> FunctionCalculateHydModel1/8(L_cyl)
  Data Store Read43/1 -> Product14/2
  [Ap] -> FunctionCalculateHydModel1/9(Aa)
  Product15/1 -> Sum10/2
  Data Store Read44/1 -> Product18/2
  Product18/1 -> Discrete-Time Integrator2/1
  [KpRl] -> Sum12/2
  [Reference] -> Sum13/2
  Constant8/1 -> FunctionCalculateHydModel1/6(Ps)
  Product14/1 -> FLcontroller1/1(pid), ScopePID1/1
  Sum11/1 -> Product16/1
  Sum12/1 -> Product15/2
  Saturation5/1 -> Divide4/1
  [Un] -> Divide4/2
  FLcontroller1/1(y) -> Product17/1
  Denormalize_Policy/1(y) -> FunctionCalculateHydModel1/15(data)
  Sum10/1 -> Product14/1
  [C1] -> FunctionCalculateHydModel1/11(c1)
  Discrete-Time Integrator2/1 -> Product16/2
  [Pn] -> FunctionCalculateHydModel1/2(Pn)
  [LastAction] -> Unit Delay/1
  [Kp] -> Sum12/1
  [Ki] -> Sum11/1
  Constant7/1 -> FunctionCalculateHydModel1/7(Pt)
  Divide4/1 -> Policy/1(u)
  [Qn] -> FunctionCalculateHydModel1/3(Qn)
  Constant3/1 -> FLcontroller1/5(d)
  [KiRl] -> Sum11/2
  Data Store Read47/1 -> Product17/2
  Product16/1 -> Sum10/1
  FunctionCalculateHydModel1/2(g) -> FLcontroller1/3(g)
  Product17/1 -> Saturation5/1
  [DReference] -> FLcontroller1/4(dFref)
  FunctionCalculateHydModel1/1(f) -> FLcontroller1/2(f)
  [Un] -> FunctionCalculateHydModel1/4(Un)
  Data Store Read46/1 -> FunctionCalculateHydModel1/14(flag_start)
  NormData/1 -> Denormalize_Policy/1(u)
  Unit Delay/1 -> FunctionCalculateHydModel1/1(ixv)
  SmoothFnc1/1(y) -> NormOut/1
  Policy/1(y) -> SmoothFnc1/1(u)
  [SmoothFactor] -> SmoothFnc1/2(smooth)
  Data Store Read19/1 -> Discrete-Time Integrator2/2

== system RealLifeTrainModel/ContractionMetricFilterSystem3/Calc_A_B/Calc_A_Grad/IndidualGrad1 ==
  State : Inport
  Position : Inport  Port=2
  StartValue : Inport  Port=3
  Data Type Conversion2 : DataTypeConversion  OutDataTypeStr=single  SaturateOnIntegerOverflow=off  RndMeth=Floor
  Data Type Conversion4 : DataTypeConversion  OutDataTypeStr=single  SaturateOnIntegerOverflow=off  RndMeth=Floor
  DynamicsConvert : MATLAB Function  TreatAsAtomicUnit=on
  MATLAB Function2 : MATLAB Function  TreatAsAtomicUnit=on
  MATLAB Function5 : MATLAB Function  TreatAsAtomicUnit=on
  Reshape : Reshape  OutputDimensionality=Customize  OutputDimensions=[8,1]
  Reshape1 : Reshape  OutputDimensionality=Customize  OutputDimensions=[8,1]
  Reshape2 : Reshape  OutputDimensionality=Customize  OutputDimensions=[8,1]
  SubsystemModel : Subsystem
  Sum4 : Sum  Inputs=|++
  Grad : Outport
  wires:
  [GradConst] -> MATLAB Function5/3(const)
  Sum4/1 -> Data Type Conversion2/1
  [GradConst] -> MATLAB Function2/1(u)
  State/1 -> Sum4/1
  MATLAB Function2/1(y) -> Sum4/2
  Position/1 -> MATLAB Function2/2(pos)
  MATLAB Function5/1(y) -> Reshape2/1
  StartValue/1 -> Reshape1/1
  Data Type Conversion2/1 -> SubsystemModel/1(u), DynamicsConvert/1(x)
  SubsystemModel/1(y) -> Data Type Conversion4/1
  [DiscreteContinousMode] -> DynamicsConvert/3(useDerivative)
  Data Type Conversion4/1 -> DynamicsConvert/2(y_model)
  DynamicsConvert/1(dstate) -> Reshape/1
  Reshape/1 -> MATLAB Function5/1(u1)
  Reshape1/1 -> MATLAB Function5/2(u2)
  Reshape2/1 -> Grad/1

== system RealLifeTrainModel/ContractionMetricFilterSystem3/Calc_A_B/Calc_A_Grad/IndidualGrad10 ==
  State : Inport
  Position : Inport  Port=2
  StartValue : Inport  Port=3
  Data Type Conversion2 : DataTypeConversion  OutDataTypeStr=single  SaturateOnIntegerOverflow=off  RndMeth=Floor
  Data Type Conversion4 : DataTypeConversion  OutDataTypeStr=single  SaturateOnIntegerOverflow=off  RndMeth=Floor
  DynamicsConvert : MATLAB Function  TreatAsAtomicUnit=on
  MATLAB Function2 : MATLAB Function  TreatAsAtomicUnit=on
  MATLAB Function5 : MATLAB Function  TreatAsAtomicUnit=on
  Reshape : Reshape  OutputDimensionality=Customize  OutputDimensions=[8,1]
  Reshape1 : Reshape  OutputDimensionality=Customize  OutputDimensions=[8,1]
  Reshape2 : Reshape  OutputDimensionality=Customize  OutputDimensions=[8,1]
  SubsystemModel : Subsystem
  Sum4 : Sum  Inputs=|++
  Grad : Outport
  wires:
  [GradConst] -> MATLAB Function5/3(const)
  Sum4/1 -> Data Type Conversion2/1
  [GradConst] -> MATLAB Function2/1(u)
  State/1 -> Sum4/1
  MATLAB Function2/1(y) -> Sum4/2
  Position/1 -> MATLAB Function2/2(pos)
  MATLAB Function5/1(y) -> Reshape2/1
  StartValue/1 -> Reshape1/1
  Data Type Conversion2/1 -> SubsystemModel/1(u), DynamicsConvert/1(x)
  SubsystemModel/1(y) -> Data Type Conversion4/1
  DynamicsConvert/1(dstate) -> Reshape/1
  Data Type Conversion4/1 -> DynamicsConvert/2(y_model)
  [DiscreteContinousMode] -> DynamicsConvert/3(useDerivative)
  Reshape/1 -> MATLAB Function5/1(u1)
  Reshape1/1 -> MATLAB Function5/2(u2)
  Reshape2/1 -> Grad/1

== system RealLifeTrainModel/ContractionMetricFilterSystem3/Calc_A_B/Calc_A_Grad/IndidualGrad2 ==
  State : Inport
  Position : Inport  Port=2
  StartValue : Inport  Port=3
  Data Type Conversion2 : DataTypeConversion  OutDataTypeStr=single  SaturateOnIntegerOverflow=off  RndMeth=Floor
  Data Type Conversion4 : DataTypeConversion  OutDataTypeStr=single  SaturateOnIntegerOverflow=off  RndMeth=Floor
  DynamicsConvert : MATLAB Function  TreatAsAtomicUnit=on
  MATLAB Function2 : MATLAB Function  TreatAsAtomicUnit=on
  MATLAB Function5 : MATLAB Function  TreatAsAtomicUnit=on
  Reshape : Reshape  OutputDimensionality=Customize  OutputDimensions=[8,1]
  Reshape1 : Reshape  OutputDimensionality=Customize  OutputDimensions=[8,1]
  Reshape2 : Reshape  OutputDimensionality=Customize  OutputDimensions=[8,1]
  SubsystemModel : Subsystem
  Sum4 : Sum  Inputs=|++
  Grad : Outport
  wires:
  [GradConst] -> MATLAB Function5/3(const)
  Sum4/1 -> Data Type Conversion2/1
  [GradConst] -> MATLAB Function2/1(u)
  State/1 -> Sum4/1
  MATLAB Function2/1(y) -> Sum4/2
  Position/1 -> MATLAB Function2/2(pos)
  MATLAB Function5/1(y) -> Reshape2/1
  StartValue/1 -> Reshape1/1
  Data Type Conversion2/1 -> SubsystemModel/1(u), DynamicsConvert/1(x)
  SubsystemModel/1(y) -> Data Type Conversion4/1
  [DiscreteContinousMode] -> DynamicsConvert/3(useDerivative)
  Data Type Conversion4/1 -> DynamicsConvert/2(y_model)
  DynamicsConvert/1(dstate) -> Reshape/1
  Reshape/1 -> MATLAB Function5/1(u1)
  Reshape1/1 -> MATLAB Function5/2(u2)
  Reshape2/1 -> Grad/1

== system RealLifeTrainModel/ContractionMetricFilterSystem3/Calc_A_B/Calc_A_Grad/IndidualGrad3 ==
  State : Inport
  Position : Inport  Port=2
  StartValue : Inport  Port=3
  Data Type Conversion2 : DataTypeConversion  OutDataTypeStr=single  SaturateOnIntegerOverflow=off  RndMeth=Floor
  Data Type Conversion4 : DataTypeConversion  OutDataTypeStr=single  SaturateOnIntegerOverflow=off  RndMeth=Floor
  DynamicsConvert : MATLAB Function  TreatAsAtomicUnit=on
  MATLAB Function2 : MATLAB Function  TreatAsAtomicUnit=on
  MATLAB Function5 : MATLAB Function  TreatAsAtomicUnit=on
  Reshape : Reshape  OutputDimensionality=Customize  OutputDimensions=[8,1]
  Reshape1 : Reshape  OutputDimensionality=Customize  OutputDimensions=[8,1]
  Reshape2 : Reshape  OutputDimensionality=Customize  OutputDimensions=[8,1]
  SubsystemModel : Subsystem
  Sum4 : Sum  Inputs=|++
  Grad : Outport
  wires:
  [GradConst] -> MATLAB Function5/3(const)
  Sum4/1 -> Data Type Conversion2/1
  [GradConst] -> MATLAB Function2/1(u)
  State/1 -> Sum4/1
  MATLAB Function2/1(y) -> Sum4/2
  Position/1 -> MATLAB Function2/2(pos)
  MATLAB Function5/1(y) -> Reshape2/1
  StartValue/1 -> Reshape1/1
  Data Type Conversion2/1 -> SubsystemModel/1(u), DynamicsConvert/1(x)
  SubsystemModel/1(y) -> Data Type Conversion4/1
  [DiscreteContinousMode] -> DynamicsConvert/3(useDerivative)
  Data Type Conversion4/1 -> DynamicsConvert/2(y_model)
  DynamicsConvert/1(dstate) -> Reshape/1
  Reshape/1 -> MATLAB Function5/1(u1)
  Reshape1/1 -> MATLAB Function5/2(u2)
  Reshape2/1 -> Grad/1

== system RealLifeTrainModel/ContractionMetricFilterSystem3/Calc_A_B/Calc_A_Grad/IndidualGrad4 ==
  State : Inport
  Position : Inport  Port=2
  StartValue : Inport  Port=3
  Data Type Conversion2 : DataTypeConversion  OutDataTypeStr=single  SaturateOnIntegerOverflow=off  RndMeth=Floor
  Data Type Conversion4 : DataTypeConversion  OutDataTypeStr=single  SaturateOnIntegerOverflow=off  RndMeth=Floor
  DynamicsConvert : MATLAB Function  TreatAsAtomicUnit=on
  MATLAB Function2 : MATLAB Function  TreatAsAtomicUnit=on
  MATLAB Function5 : MATLAB Function  TreatAsAtomicUnit=on
  Reshape : Reshape  OutputDimensionality=Customize  OutputDimensions=[8,1]
  Reshape1 : Reshape  OutputDimensionality=Customize  OutputDimensions=[8,1]
  Reshape2 : Reshape  OutputDimensionality=Customize  OutputDimensions=[8,1]
  SubsystemModel : Subsystem
  Sum4 : Sum  Inputs=|++
  Grad : Outport
  wires:
  [GradConst] -> MATLAB Function5/3(const)
  Sum4/1 -> Data Type Conversion2/1
  [GradConst] -> MATLAB Function2/1(u)
  State/1 -> Sum4/1
  MATLAB Function2/1(y) -> Sum4/2
  Position/1 -> MATLAB Function2/2(pos)
  MATLAB Function5/1(y) -> Reshape2/1
  StartValue/1 -> Reshape1/1
  Data Type Conversion2/1 -> SubsystemModel/1(u), DynamicsConvert/1(x)
  SubsystemModel/1(y) -> Data Type Conversion4/1
  [DiscreteContinousMode] -> DynamicsConvert/3(useDerivative)
  Data Type Conversion4/1 -> DynamicsConvert/2(y_model)
  DynamicsConvert/1(dstate) -> Reshape/1
  Reshape/1 -> MATLAB Function5/1(u1)
  Reshape1/1 -> MATLAB Function5/2(u2)
  Reshape2/1 -> Grad/1

== system RealLifeTrainModel/ContractionMetricFilterSystem3/Calc_A_B/Calc_A_Grad/IndidualGrad5 ==
  State : Inport
  Position : Inport  Port=2
  StartValue : Inport  Port=3
  Data Type Conversion2 : DataTypeConversion  OutDataTypeStr=single  SaturateOnIntegerOverflow=off  RndMeth=Floor
  Data Type Conversion4 : DataTypeConversion  OutDataTypeStr=single  SaturateOnIntegerOverflow=off  RndMeth=Floor
  DynamicsConvert : MATLAB Function  TreatAsAtomicUnit=on
  MATLAB Function2 : MATLAB Function  TreatAsAtomicUnit=on
  MATLAB Function5 : MATLAB Function  TreatAsAtomicUnit=on
  Reshape : Reshape  OutputDimensionality=Customize  OutputDimensions=[8,1]
  Reshape1 : Reshape  OutputDimensionality=Customize  OutputDimensions=[8,1]
  Reshape2 : Reshape  OutputDimensionality=Customize  OutputDimensions=[8,1]
  SubsystemModel : Subsystem
  Sum4 : Sum  Inputs=|++
  Grad : Outport
  wires:
  [GradConst] -> MATLAB Function5/3(const)
  Sum4/1 -> Data Type Conversion2/1
  [GradConst] -> MATLAB Function2/1(u)
  State/1 -> Sum4/1
  MATLAB Function2/1(y) -> Sum4/2
  Position/1 -> MATLAB Function2/2(pos)
  MATLAB Function5/1(y) -> Reshape2/1
  StartValue/1 -> Reshape1/1
  Data Type Conversion2/1 -> SubsystemModel/1(u), DynamicsConvert/1(x)
  SubsystemModel/1(y) -> Data Type Conversion4/1
  [DiscreteContinousMode] -> DynamicsConvert/3(useDerivative)
  Data Type Conversion4/1 -> DynamicsConvert/2(y_model)
  DynamicsConvert/1(dstate) -> Reshape/1
  Reshape/1 -> MATLAB Function5/1(u1)
  Reshape1/1 -> MATLAB Function5/2(u2)
  Reshape2/1 -> Grad/1
